simulink model "cuirtuitb2"  (R2022b)
settings: Solver=VariableStepAuto  StartTime=0.0  StopTime=10.0  RelTol=1e-3
settings Model: Creator=Paulo Cortesão  LastModifiedBy=Paulo Cortesão

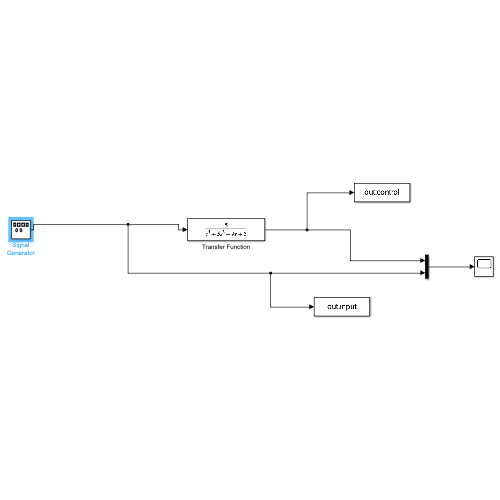
[thumbnail: Simulink's stored preview of the top-level diagram]
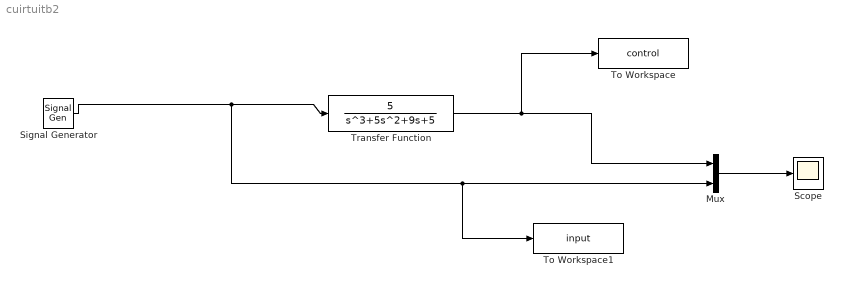
== system cuirtuitb2 ==
  Mux : Mux  Inputs=2
  Scope : Scope
  Signal Generator : SignalGenerator  WaveForm=random  Frequency=0.01  Units=rad/sec
  To Workspace : ToWorkspace  VariableName=control  SaveFormat=Timeseries  SampleTime=-1
  To Workspace1 : ToWorkspace  VariableName=input  SaveFormat=Timeseries  SampleTime=-1
  Transfer Function : TransferFcn  Numerator=[5]  Denominator=[1 5 9 5]
  wires:
  Mux/1 -> Scope/1
  Transfer Function/1 -> To Workspace/1, Mux/1
  Signal Generator/1 -> To Workspace1/1, Mux/2, Transfer Function/1
